simulink model "BESS_test_new"  (Simulink 8.1)
settings: Solver=ode1  StartTime=0.0  StopTime=15  FixedStep=Ts  MaxStep=1e-3  RelTol=1e-3
model workspace (MAT data in the model file):
  op_snapshot1 : opcond.OperatingPoint (value not decoded)
undefined symbols (not defined in the file or in its folder): f, H, Lgrid, Pgrid, Rgrid, RotatingMachine_lib, sampdT, sys_mech, Tc, Ts, Vgrid, VSource
libraries: powerlib x26, powerlib_meascontrol x6, transformer_lib x4, simulink x4, breaker_lib x3, Load_lib x3, cables_lib x2, BESS_lib x1, debounce_lib x1
settings Model: ARTEMISmethode_block_infos=$$__separator__$$RS/ARTEMIS Guide$$__separator__$$  Creator=RE25624  LastModifiedBy=ch24070  SimulationMode=accelerator
settings SolverCC: ZeroCrossAlgorithm=Adaptive
settings DataIOCC: ExternalInput=getinputstruct(op_snapshot1)  InitialState=getstatestruct(op_snapshot1)  LimitDataPoints=off  MaxDataPoints=90060  SignalLoggingSaveFormat=Dataset  SaveOutput=off  SignalLogging=off  DSMLogging=off  SaveTime=off  OutputSaveName=result
settings OptimizationCC: BlockReduction=off  OptimizeBlockIOStorage=off  BufferReuse=off  ExpressionFolding=off  LocalBlockOutputs=off  EfficientMapNaN2IntZero=off
settings DebuggingCC: MaxConsecutiveZCsMsg=warning  IgnoredZcDiagnostic=none  SolverPrmCheckMsg=none  MultiTaskRateTransMsg=warning  FcnCallInpInsideContextMsg=EnableAllAsWarning  UnconnectedLineMsg=none  FrameProcessingCompatibilityMsg=error  ModelReferenceExtraNoncontSigs=warning
settings HardwareCC: TargetBitPerPointer=64  TargetLongLongMode=on  TargetIntDivRoundTo=Zero  TargetEndianess=LittleEndian  TargetWordSize=64  TargetHWDeviceType=MATLAB Host  ProdEqTarget=off
settings ModelReferenceCC: UpdateModelReferenceTargets=IfOutOfDate
settings SFSimCC: SFSimEcho=off
settings CodeAppCC: MaxIdLength=128
settings GRTTargetCC: CodeReplacementLibrary=C89/C90 (ANSI)  GeneratePreprocessorConditionals=Use local settings

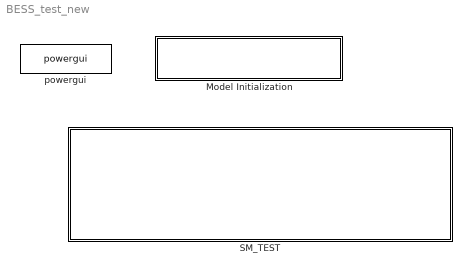
== system BESS_test_new ==
  Model Initialization : Subsystem  AncestorBlock=artemis/Tools /Misc/Model Initialization  mask(Model Functions){InitFcnX=, prel=off, posl=on, inif=on, strf=off}
      mask prompts: InitFcnX "Initialisation"; prel "Preload Function"; posl "PostLoad Function"; inif "InitFcn"; strf "StartFcn"
      mask init:
      | currentBlock = gcb;
      | root = bdroot(currentBlock);
      | 
      | if ~strcmp(get_param(root,'BlockDiagramType'),'library')
      |     if prel==1
      |         set_param(root, 'PreLoadFcn', InitFcnX);
      |     else
      |         set_param(root, 'PreLoadFcn', '');
      |     end
      |     if inif==1
      |         set_param(root, 'InitFcn', InitFcnX);
      |     else
      |         set_param(root, 'InitFcn', '');
      |     end
      |     if strf==1
      |         set_param(root, 'StartFcn', InitFcnX);
      |     else
      |         set_param(root, 'StartFcn', '');
      |     end
      |     if posl==1
      |         set_param(root, 'PostLoadFcn', InitFcnX);
      |     else
      |         set_param(root, 'PostLoadFcn', '');
      |     end
      | end
      | 
      | pos = get_param(currentBlock, 'Position');
      | width = pos(3) - pos(1); height = pos(4) - pos(2);
      | txt = [ upper(root) '\n' '- InitFcn. . . . . '  get_param(root, 'InitFcn') ];
      settings: CopyFcn=set_param(gcb,'LinkStatus','inactive')
      mask Display: text(5, height*0.5, txt, 'horizontalAlignment', 'left', 'verticalAlignment', 'middle') ;
  SM_TEST : Subsystem
  powergui : powerlib/powergui  Priority=2  SimulationMode=Discrete  SolverType=Tustin  SampleTime=Ts  frequency=60  SPID=off  DisableSnubberDevices=off  DisableRonSwitches=off  DisableVfSwitches=off  SwTol=0  DisplayEquations=off  Interpol=off  ExternalGateDelay=off  methode=off  Ts=0  FunctionMessages=off  echomessages=off  HookPort=off  EnableUseOfTLC=off  x0status=blocks  frequencyindice=0  Pbase=100e6  ErrMax=1e-4  Iterations=50  UnitsV=kV  UnitsW=MW  buscounter=0  RestoreLinks=warning  ResistiveCurrentMeasurement=off  Frange=logspace(-2,3,50)  Ylog=on  Xlog=on  ShowGrid=off  save=off  variable=ZData  structure=0  ZoomFFT=on  StartTime=0.0  cycles=2  DisplayStyle=off  fundamental=60  FreqAxis=off  MaxFrequency=1000  frequencyindicesteady=1  RmsSteady=1  display=off

== system BESS_test_new/Model Initialization ==

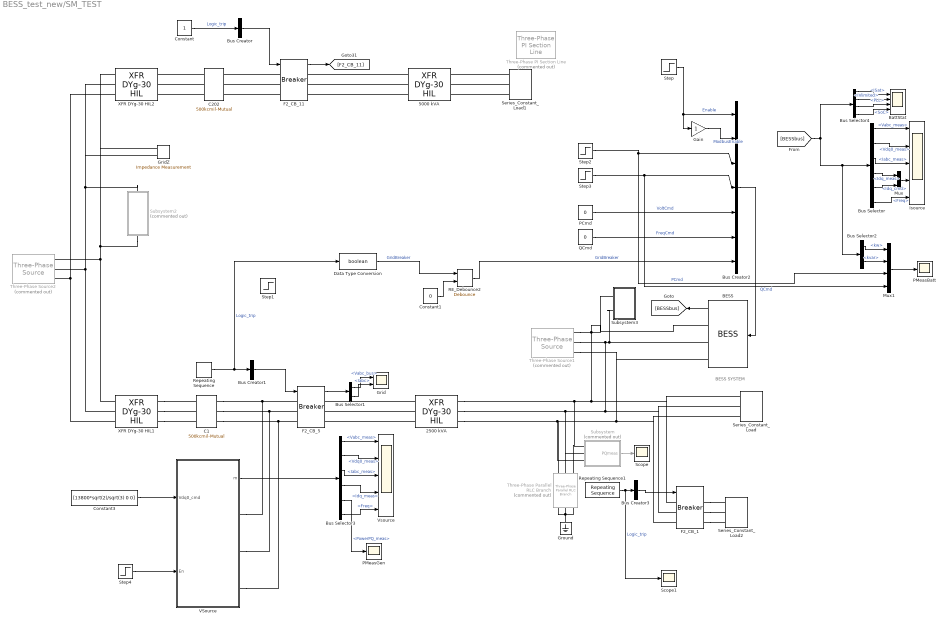
== system BESS_test_new/SM_TEST ==
  note: BESS SYSTEM
  2500 kVA : transformer_lib/XFR DYg-30 HIL  Rating=2500  Vp=13800  Vs=480  Z=5.56  XR=5.52
  5000 kVA : transformer_lib/XFR DYg-30 HIL  Rating=5000  Vp=13800  Vs=480  Z=5.50  XR=5.44
  BESS : BESS_lib/BESS
  BattStat : Scope  NumInputPorts=4
      settings: TimeRange=auto  MaxDataPoints=5000  SaveToWorkspace=off  SaveName=ScopeData2  YMin=-1.00000~-1.00000~-0.125~49.999925  YMax=1.00000~1.00000~1.125~50.000008  SampleTime=-1
  Bus Creator : BusCreator  Inputs=1
  Bus Creator1 : BusCreator  Inputs=1
  Bus Creator2 : BusCreator  Inputs=7
  Bus Creator3 : BusCreator  Inputs=1
  Bus Selector : BusSelector  OutputSignals=Inverter.Vabc_meas,Inverter.Vdq0_meas,Inverter.Iabc_meas,Inverter.Idq_meas,Inverter.Idq_cmd,Inverter.Freq
  Bus Selector1 : BusSelector  OutputSignals=Vabc_bus,Iabc
  Bus Selector2 : BusSelector  OutputSignals=Inverter.kw,Inverter.kvar
  Bus Selector3 : BusSelector  OutputSignals=Vabc_meas,Vdq0_meas,Iabc_meas,Idq_meas,PowerPQ_meas,Freq
  Bus Selector4 : BusSelector  OutputSignals=Inverter.faults.ISat,Inverter.faults.IVlimited,Inverter.faults.PLL,Battery.SoC
  C1 : cables_lib/500kcmil-Mutual  length=2000  par_sets=1  ratio=3
  C202 : cables_lib/500kcmil-Mutual  length=2000  par_sets=1  ratio=3
  Constant : Constant
  Constant1 : Constant  Value=0
  Constant3 : Constant  Value=[13800*sqrt(2)/sqrt(3) 0 0]
  Data Type Conversion : DataTypeConversion  OutDataTypeStr=boolean
  F2_CB_1 : breaker_lib/Breaker  Ts=Ts  mech_delay=3/60
  F2_CB_11 : breaker_lib/Breaker  Ts=Ts  mech_delay=3/60
  F2_CB_5 : breaker_lib/Breaker  Ts=Ts  mech_delay=3/60
  Gain : Gain
  Grid : Scope  NumInputPorts=2
      settings: TimeRange=auto  MaxDataPoints=5000  SaveToWorkspace=off  SaveName=ScopeData2  YMin=-14548.7743~-76.73519  YMax=14146.20278~74.89717  SampleTime=-1
  GridZ : powerlib/Measurements/Impedance Measurement  LConnTagsString=+|-  Factor=1
  Ground : powerlib/Elements/Ground  LConnTagsString=a
  Isource : Scope  NumInputPorts=5
      settings: TimeRange=auto  MaxDataPoints=5000  SaveName=ScopeData  YMin=-637.83955~-497.79073~-1602.05268~-1092.74993~59.90896  YMax=586.43964~568.58935~1602.13671~1545.94373~60.13357  SampleTime=-1
  Mux : Mux  Inputs=2
  Mux1 : Mux
  PCmd : Constant  Value=0
  PMeasBatt : Scope
      settings: TimeRange=auto  MaxDataPoints=5000  SaveToWorkspace=off  YMin=-1678.43829  YMax=1001.5492  SampleTime=-1
  PMeasGen : Scope
      settings: TimeRange=auto  MaxDataPoints=5000  SaveToWorkspace=off  SaveName=ScopeData2  YMin=-2639050.74714  YMax=4701504.7437  SampleTime=-1
  QCmd : Constant  Value=0
  RE_Debounce2 : debounce_lib/Debounce  Ts=sampdT  Td=0.05
  Repeating Sequence : simulink/Sources/Repeating Sequence  rep_seq_t=[0 2 2+Ts 6 6+Ts 100]  rep_seq_y=[1 1 0 0 1 1]
  Repeating Sequence1 : simulink/Sources/Repeating Sequence  rep_seq_t=[0, 4, 4+Ts, 5, 5+Ts, 8, 8+Ts 20]  rep_seq_y=[0 0 1 1 0 0 1 1]
  Scope : Scope
      settings: TimeRange=auto  MaxDataPoints=5000  SaveToWorkspace=off  YMin=-798029.94386  YMax=1422067.88409  SampleTime=-1
  Scope1 : Scope
      settings: TimeRange=auto  MaxDataPoints=5000  SaveToWorkspace=off  SaveName=ScopeData3  YMin=-0.125  YMax=1.125  SampleTime=-1
  Series_Constant_Load : Load_lib/Series_Constant_Load  v=460  kVA=400  pf=0.90
  Series_Constant_Load1 : Load_lib/Series_Constant_Load  v=460  kVA=100  pf=0.90
  Series_Constant_Load2 : Load_lib/Series_Constant_Load  v=460  kVA=300  pf=0.90
  Step : Step  Time=0.1  SampleTime=0
  Step1 : Step  Time=0.5  Before=1  After=0  SampleTime=0
  Step2 : Step  Time=13.5  After=-500  SampleTime=0
  Step3 : Step  Time=14  After=-500  SampleTime=0
  Step4 : Step  Time=0  SampleTime=0
  Subsystem : Subsystem  Commented=on  mask{V=480, P=1e3, PF=0.9}
      mask prompts: V "Nominal voltage LL"; P "P (kVA)"
      mask init:
      | Rpar = V^2/(P*1e3*PF)
      | Lpar = (V^2/((P*1e3*sqrt(1-PF^2))/3))/377
      | if Lpar == Inf
      |     Lser=0
      |     Rser=Rpar
      | else
      |     Lser = 1e-3
      |     Rser = (-Lpar^2)/(Rpar+Lpar)+Lpar-Lser
      | end
  Subsystem2 : Subsystem  Commented=on
  Subsystem3 : Subsystem
  Three-Phase PI Section Line : powerlib/Elements/Three-Phase PI Section Line  Commented=on  LConnTagsString=a|b|c  RConnTagsString=A|B|C  Frequency=60  Resistances=[ 0.01273 0.3864]  Inductances="[ 0.9337e-3  4.1264e-3]"  Capacitances=[12.74e-9 7.751e-9]  Length=100
  Three-Phase Parallel RLC Branch : powerlib/Elements/Three-Phase Parallel RLC Branch  Commented=on  LConnTagsString=A|B|C  RConnTagsString=A|B|C  BranchType=R  Resistance=Vgrid^2/(200*1e3/3);  Inductance=(Vgrid^2/((1000e3*sqrt(1-0.9^2))/3))/377  Capacitance=1e-6  Measurements=None
  Three-Phase Source1 : powerlib/Electrical Sources/Three-Phase Source  Commented=on  InternalConnection=Yg  VoltagePhases=off  Voltage=480  PhaseAngle=0  Voltage_phases=[25e3 25e3 25e3]/sqrt(3)  PhaseAngles_phases=[0 -120 +120]  Frequency=60  NonIdealSource=on  SpecifyImpedance=off  Resistance=Lgrid  Inductance=Rgrid  ShortCircuitLevel=2000e6  BaseVoltage=480  XRratio=100  BusType=swing  Pref=0  Qref=0  Prefabc=[10e3, 10e3, 10e3]  Qrefabc=[0, 0, 0]  Qmin=-inf  Qmax=inf
  Three-Phase Source2 : powerlib/Electrical Sources/Three-Phase Source  Commented=on  InternalConnection=Yg  VoltagePhases=off  Voltage=115000  PhaseAngle=0  Voltage_phases=[25e3 25e3 25e3]/sqrt(3)  PhaseAngles_phases=[0 -120 +120]  Frequency=60  NonIdealSource=on  SpecifyImpedance=on  Resistance=0.8929  Inductance=16.58e-3  ShortCircuitLevel=2000e6  BaseVoltage=115000  XRratio=100  BusType=swing  Pref=0  Qref=0  Prefabc=[10e3, 10e3, 10e3]  Qrefabc=[0, 0, 0]  Qmin=-inf  Qmax=inf
  VSource : Subsystem  AncestorBlock=RotatingMachine_lib/VSource
  Vsource : Scope  NumInputPorts=5
      settings: TimeRange=auto  MaxDataPoints=5000  YMin=-14095.34302~-1426.98059~-258.17624~-157.47216~59.97105  YMax=14085.47927~12733.83164~249.33503~278.13701~60.01653  SampleTime=-1
  XFR DYg-30 HIL1 : transformer_lib/XFR DYg-30 HIL  Rating=50000  Vp=115000  Vs=13800  Z=6  XR=30
  XFR DYg-30 HIL2 : transformer_lib/XFR DYg-30 HIL  Rating=50000  Vp=115000  Vs=13800  Z=6  XR=30
  wires:
  F2_CB_5/1 -> Bus Selector1/1
  F2_CB_11/1 -> [F2_CB_11]
  Constant/1 -> Bus Creator/1  "Logic_trip"
  Repeating Sequence/1 -> Data Type Conversion/1, Bus Creator1/1  "Logic_trip"
  Bus Creator1/1 -> F2_CB_5/1
  Bus Creator/1 -> F2_CB_11/1
  Step/1 -> Gain/1, Bus Creator2/1  "Enable"
  Step2/1 -> Mux1/3, Bus Creator2/3  "PCmd"
  Step3/1 -> Mux1/4, Bus Creator2/4  "QCmd"
  Bus Creator2/1 -> BESS/1
  Bus Selector/6 -> Isource/5  "<Freq>"
  Bus Selector/3 -> Isource/3  "<Iabc_meas>"
  Bus Selector/1 -> Isource/1  "<Vabc_meas>"
  Bus Selector/2 -> Isource/2  "<Vdq0_meas>"
  Subsystem/1(PQmeas) -> Scope/1
  Bus Selector1/1 -> Grid/1  "<Vabc_bus>"
  Bus Selector1/2 -> Grid/2  "<Iabc>"
  Mux/1 -> Isource/4
  Bus Selector/4 -> Mux/1  "<Idq_meas>"
  Bus Selector/5 -> Mux/2  "<Idq_cmd>"
  BESS/1 -> [BESSbus]
  [BESSbus] -> Bus Selector/1, Bus Selector2/1, Bus Selector4/1
  Bus Selector2/1 -> Mux1/1  "<kw>"
  Mux1/1 -> PMeasBatt/1
  Repeating Sequence1/1 -> Scope1/1, Bus Creator3/1  "Logic_trip"
  Bus Creator3/1 -> F2_CB_1/1
  Constant3/1 -> VSource/1(Vdq0_cmd)
  Step4/1 -> VSource/2(En)
  Bus Selector3/3 -> Vsource/3  "<Iabc_meas>"
  Bus Selector3/1 -> Vsource/1  "<Vabc_meas>"
  Bus Selector3/2 -> Vsource/2  "<Vdq0_meas>"
  Bus Selector3/4 -> Vsource/4  "<Idq_meas>"
  VSource/1(m) -> Bus Selector3/1
  Bus Selector3/6 -> Vsource/5  "<Freq>"
  Bus Selector3/5 -> PMeasGen/1  "<PowerPQ_meas>"
  Gain/1 -> Bus Creator2/2  "ModbusEnable"
  Bus Selector2/2 -> Mux1/2  "<kvar>"
  Bus Selector4/2 -> BattStat/2  "<IVlimited>"
  Bus Selector4/1 -> BattStat/1  "<ISat>"
  Bus Selector4/3 -> BattStat/3  "<PLL>"
  PCmd/1 -> Bus Creator2/5  "VoltCmd"
  QCmd/1 -> Bus Creator2/6  "FreqCmd"
  RE_Debounce2/1 -> Bus Creator2/7  "GridBreaker"
  Bus Selector4/4 -> BattStat/4  "<SoC>"
  Constant1/1 -> RE_Debounce2/2
  Data Type Conversion/1 -> RE_Debounce2/1  "GridBreaker"
  connections:
  5000 kVA/LConn2 -- F2_CB_11/RConn2
  2500 kVA/LConn1 -- F2_CB_5/RConn1
  2500 kVA/LConn3 -- F2_CB_5/RConn3
  2500 kVA/LConn2 -- F2_CB_5/RConn2
  5000 kVA/LConn1 -- F2_CB_11/RConn1
  5000 kVA/LConn3 -- F2_CB_11/RConn3
  2500 kVA/RConn1 -- BESS/RConn1 -- Subsystem3/LConn1 -- Three-Phase Source1/RConn1 -- F2_CB_1/LConn1 -- Series_Constant_Load/LConn1 -- Three-Phase Parallel RLC Branch/LConn3 -- Subsystem/LConn1
  2500 kVA/RConn3 -- BESS/RConn3 -- Three-Phase Source1/RConn3 -- F2_CB_1/LConn3 -- Series_Constant_Load/LConn3 -- Three-Phase Parallel RLC Branch/LConn1 -- Subsystem/LConn3
  XFR DYg-30 HIL1/LConn1 -- GridZ/LConn1 -- XFR DYg-30 HIL2/LConn1 -- Subsystem2/LConn1 -- Three-Phase Source2/RConn1
  XFR DYg-30 HIL1/LConn2 -- GridZ/LConn2 -- XFR DYg-30 HIL2/LConn2 -- Subsystem2/RConn1 -- Three-Phase Source2/RConn2
  XFR DYg-30 HIL1/LConn3 -- XFR DYg-30 HIL2/LConn3 -- Three-Phase Source2/RConn3
  Series_Constant_Load1/LConn3 -- 5000 kVA/RConn3
  Series_Constant_Load1/LConn2 -- 5000 kVA/RConn2
  Series_Constant_Load1/LConn1 -- 5000 kVA/RConn1
  C202/LConn1 -- XFR DYg-30 HIL2/RConn1
  C202/LConn2 -- XFR DYg-30 HIL2/RConn2
  C202/LConn3 -- XFR DYg-30 HIL2/RConn3
  XFR DYg-30 HIL1/RConn1 -- C1/LConn1
  XFR DYg-30 HIL1/RConn2 -- C1/LConn2
  XFR DYg-30 HIL1/RConn3 -- C1/LConn3
  C1/RConn2 -- VSource/RConn2 -- F2_CB_5/LConn2
  C1/RConn1 -- VSource/RConn1 -- F2_CB_5/LConn1
  C1/RConn3 -- VSource/RConn3 -- F2_CB_5/LConn3
  F2_CB_11/LConn1 -- C202/RConn1
  F2_CB_11/LConn2 -- C202/RConn2
  F2_CB_11/LConn3 -- C202/RConn3
  Ground/LConn1 -- Three-Phase Parallel RLC Branch/RConn3 -- Three-Phase Parallel RLC Branch/RConn1 -- Three-Phase Parallel RLC Branch/RConn2
  F2_CB_1/RConn1 -- Series_Constant_Load2/LConn1
  F2_CB_1/RConn2 -- Series_Constant_Load2/LConn2
  F2_CB_1/RConn3 -- Series_Constant_Load2/LConn3
  Subsystem3/LConn2 -- BESS/RConn2 -- 2500 kVA/RConn2 -- Three-Phase Parallel RLC Branch/LConn2 -- Subsystem/LConn2 -- F2_CB_1/LConn2 -- Series_Constant_Load/LConn2 -- Three-Phase Source1/RConn2

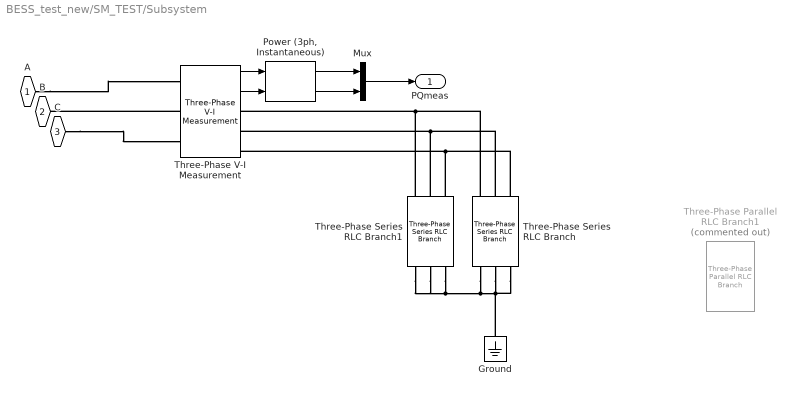
== system BESS_test_new/SM_TEST/Subsystem ==
  Ground : powerlib/Elements/Ground  LConnTagsString=a
  Mux : Mux  Inputs=2
  "Power (3ph, Instantaneous)" : powerlib_meascontrol/Measurements/Power (3ph, Instantaneous)
  Three-Phase Parallel RLC Branch1 : powerlib/Elements/Three-Phase Parallel RLC Branch  Commented=on  LConnTagsString=A|B|C  RConnTagsString=A|B|C  BranchType=RL  Resistance=Vgrid^2/(1000e3*0.9/3)  Inductance=(Vgrid^2/((1000e3*sqrt(1-0.9^2))/3))/377  Capacitance=1e-6  Measurements=None
  Three-Phase Series RLC Branch : powerlib/Elements/Three-Phase Series RLC Branch  LConnTagsString=A|B|C  RConnTagsString=A|B|C  BranchType=L  Resistance=Rser  Inductance=Lpar  Capacitance=1e-6  Measurements=None
  Three-Phase Series RLC Branch1 : powerlib/Elements/Three-Phase Series RLC Branch  LConnTagsString=A|B|C  RConnTagsString=A|B|C  BranchType=R  Resistance=Rpar  Inductance=Lser  Capacitance=1e-6  Measurements=None
  Three-Phase V-I Measurement : powerlib/Measurements/Three-Phase V-I Measurement  VoltageMeasurement=phase-to-ground  SetLabelV=off  LabelV=Vabc  Vpu=off  VpuLL=off  CurrentMeasurement=yes  SetLabelI=off  LabelI=Iabc  Ipu=off  Pbase=100e6  Vbase=500e3  OutputType=Complex  PhasorSimulation=off  PSBequivalent=0
  A : PMIOPort  Port=1  Side=Left
  B : PMIOPort  Port=2  Side=Left
  C : PMIOPort  Port=3  Side=Left
  PQmeas : Outport
  wires:
  Three-Phase V-I Measurement/1 -> "Power (3ph, Instantaneous)"/1
  Three-Phase V-I Measurement/2 -> "Power (3ph, Instantaneous)"/2
  "Power (3ph, Instantaneous)"/1 -> Mux/1
  "Power (3ph, Instantaneous)"/2 -> Mux/2
  Mux/1 -> PQmeas/1
  connections:
  Three-Phase V-I Measurement/LConn2 -- B/RConn1
  C/RConn1 -- Three-Phase V-I Measurement/LConn3
  A/RConn1 -- Three-Phase V-I Measurement/LConn1
  Three-Phase Series RLC Branch/LConn1 -- Three-Phase Series RLC Branch1/LConn1 -- Three-Phase V-I Measurement/RConn1
  Three-Phase Series RLC Branch/LConn2 -- Three-Phase Series RLC Branch1/LConn2 -- Three-Phase V-I Measurement/RConn2
  Three-Phase Series RLC Branch/LConn3 -- Three-Phase Series RLC Branch1/LConn3 -- Three-Phase V-I Measurement/RConn3
  Ground/LConn1 -- Three-Phase Series RLC Branch1/RConn3 -- Three-Phase Series RLC Branch1/RConn2 -- Three-Phase Series RLC Branch1/RConn1 -- Three-Phase Series RLC Branch/RConn1 -- Three-Phase Series RLC Branch/RConn2 -- Three-Phase Series RLC Branch/RConn3

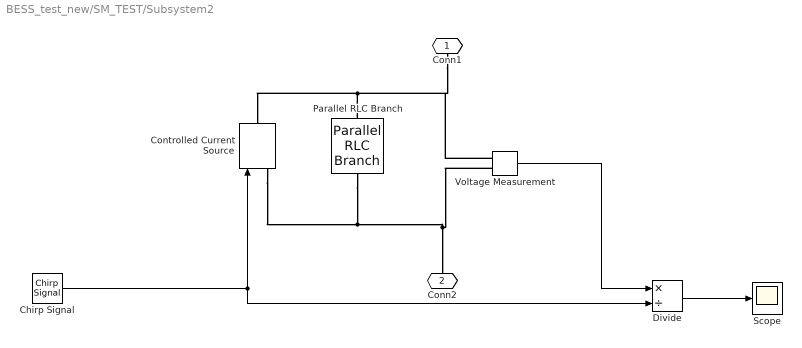
== system BESS_test_new/SM_TEST/Subsystem2 ==
  Chirp Signal : simulink/Sources/Chirp Signal  f1=0.1  T=1  f2=1000
  Controlled Current Source : powerlib/Electrical Sources/Controlled Current Source  Initialize=on  Source_Type=AC  Amplitude=0  Phase=0  Frequency=0  Measurements=None
  Divide : Product  Inputs=*/
  Parallel RLC Branch : powerlib/Elements/Parallel RLC Branch  LConnTagsString=a  RConnTagsString=__new0  BranchType=R  Resistance=1e6  Inductance=1e-3  SetiL0=off  InitialCurrent=0  Capacitance=1e-6  Setx0=off  InitialVoltage=0  Measurements=None
  Scope : Scope
      settings: TimeRange=auto  MaxDataPoints=5000  SaveToWorkspace=off  YMin=-88482354.99366  YMax=99069686.1974  SampleTime=-1
  Voltage Measurement : powerlib/Measurements/Voltage Measurement  PhasorSimulation=off  OutputType=Complex  PSBequivalent=0
  Conn1 : PMIOPort  Port=1  Side=Right
  Conn2 : PMIOPort  Port=2  Side=Left
  wires:
  Chirp Signal/1 -> Divide/2, Controlled Current Source/1
  Voltage Measurement/1 -> Divide/1
  Divide/1 -> Scope/1
  connections:
  Controlled Current Source/LConn1 -- Parallel RLC Branch/RConn1 -- Voltage Measurement/LConn2 -- Conn2/RConn1
  Parallel RLC Branch/LConn1 -- Conn1/RConn1 -- Voltage Measurement/LConn1 -- Controlled Current Source/RConn1

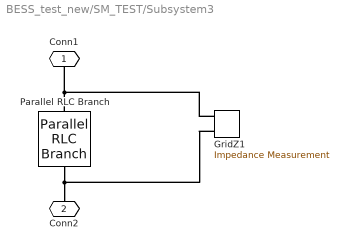
== system BESS_test_new/SM_TEST/Subsystem3 ==
  GridZ1 : powerlib/Measurements/Impedance Measurement  LConnTagsString=+|-  Factor=1
  Parallel RLC Branch : powerlib/Elements/Parallel RLC Branch  LConnTagsString=a  RConnTagsString=__new0  BranchType=R  Resistance=1e6  Inductance=1e-3  SetiL0=off  InitialCurrent=0  Capacitance=1e-6  Setx0=off  InitialVoltage=0  Measurements=None
  Conn1 : PMIOPort  Port=1  Side=Left
  Conn2 : PMIOPort  Port=2  Side=Left
  connections:
  GridZ1/LConn1 -- Parallel RLC Branch/LConn1 -- Conn1/RConn1
  GridZ1/LConn2 -- Parallel RLC Branch/RConn1 -- Conn2/RConn1

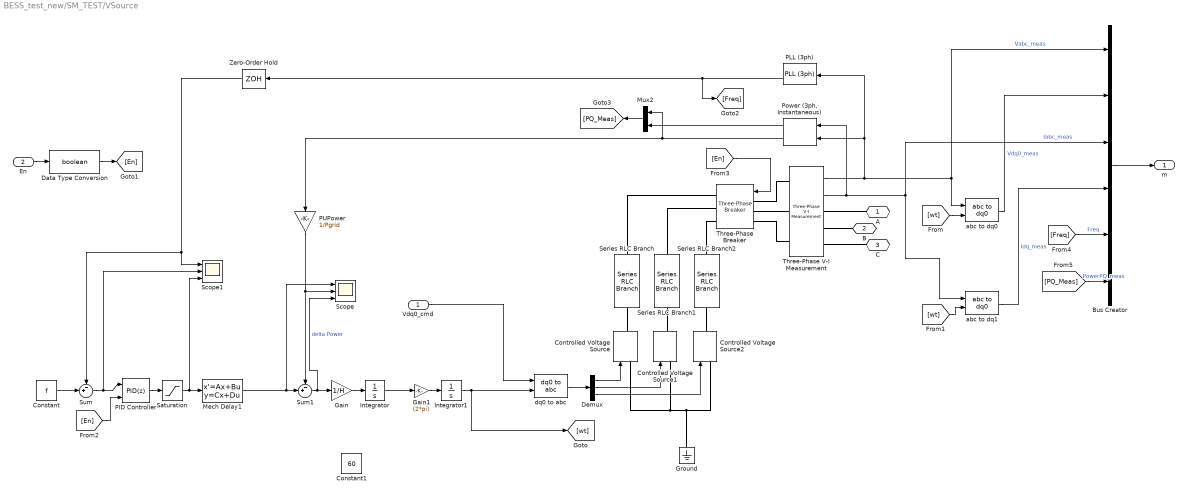
== system BESS_test_new/SM_TEST/VSource ==
  Vdq0_cmd : Inport
  En : Inport  Port=2
  Bus Creator : BusCreator  Inputs=6
  Constant : Constant  Value=f
  Constant1 : Constant  Value=60
  Controlled Voltage Source : powerlib/Electrical Sources/Controlled Voltage Source  Initialize=on  Source_Type=AC  Amplitude=0  Phase=0  Frequency=0  Measurements=None
  Controlled Voltage Source1 : powerlib/Electrical Sources/Controlled Voltage Source  Initialize=on  Source_Type=AC  Amplitude=0  Phase=0  Frequency=0  Measurements=None
  Controlled Voltage Source2 : powerlib/Electrical Sources/Controlled Voltage Source  Initialize=on  Source_Type=AC  Amplitude=0  Phase=0  Frequency=0  Measurements=None
  Data Type Conversion : DataTypeConversion  OutDataTypeStr=boolean
  Demux : Demux  Outputs=3
  Gain : Gain  Gain=1/H
  Gain1 : Gain  Gain=(2*pi)
  Ground : powerlib/Elements/Ground  LConnTagsString=a
  Integrator : Integrator  InitialCondition=f
  Integrator1 : Integrator
  Mech Delay1 : StateSpace  A=sys_mech.A  B=sys_mech.B  C=sys_mech.C  D=sys_mech.D  X0=0.3/sys_mech.C
  Mux2 : Mux  Inputs=2
  PID Controller : simulink/Continuous/PID Controller  Controller=PID  TimeDomain=Discrete-time  SampleTime=Tc  IntegratorMethod=Forward Euler  FilterMethod=Forward Euler  Form=Parallel  UseFilter=on  ControllerParametersSource=internal  P=10.7070638462033  I=6.52954426447568  D=2.34676955636377  N=24.9126202349528  InitialConditionSource=internal  InitialConditionForIntegrator=0.1  InitialConditionForFilter=0  ExternalReset=level  LimitOutput=off  UpperSaturationLimit=inf  LowerSaturationLimit=-inf  LinearizeAsGain=on  AntiWindupMode=none  Kb=1  TrackingMode=off  Kt=1  PParamMin=[]  PParamMax=[]  IParamMin=[]  IParamMax=[]  DParamMin=[]  DParamMax=[]  NParamMin=[]  NParamMax=[]  KbParamMin=[]  KbParamMax=[]  KtParamMin=[]  KtParamMax=[]  POutMin=[]  POutMax=[]  IOutMin=[]  IOutMax=[]  DOutMin=[]  DOutMax=[]  NOutMin=[]  NOutMax=[]  KbOutMin=[]  KbOutMax=[]  KtOutMin=[]  KtOutMax=[]  IntegratorOutMin=[]  IntegratorOutMax=[]  FilterOutMin=[]  FilterOutMax=[]  SumOutMin=[]  SumOutMax=[]  SumI1OutMin=[]  SumI1OutMax=[]  SumI2OutMin=[]  SumI2OutMax=[]  SumI3OutMin=[]  SumI3OutMax=[]  SumDOutMin=[]  SumDOutMax=[]  SaturationOutMin=[]  SaturationOutMax=[]  IntegratorContinuousStateAttributes=''  IntegratorStateMustResolveToSignalObject=off  IntegratorRTWStateStorageClass=Auto  FilterContinuousStateAttributes=''  FilterStateMustResolveToSignalObject=off  FilterRTWStateStorageClass=Auto  DifferentiatorICPrevScaledInput=0  DifferentiatorOutMin=[]  DifferentiatorOutMax=[]
  PLL (3ph) : powerlib_meascontrol/PLL/PLL (3ph)  Fmin=45  Par_Init=[0, 60]  ParK=[180, 3200, 1]  TcD=1e-4  MaxRateChangeFreq=1200  FilterCutOffFreq=25  Ts=0  AGC=on
  PUPower : Gain  Gain=1/Pgrid
  "Power (3ph, Instantaneous)" : powerlib_meascontrol/Measurements/Power (3ph, Instantaneous)
  Saturation : Saturate  UpperLimit=1.2  LowerLimit=0
  Scope : Scope  NumInputPorts=3
      settings: TimeRange=auto  MaxDataPoints=5000  SaveToWorkspace=off  SaveName=ScopeData3  YMin=0.0899~-0.60777~-5.51951  YMax=0.32334~5.65357~0.78328  SampleTime=-1
  Scope1 : Scope  NumInputPorts=3
      settings: TimeRange=auto  MaxDataPoints=5000  SaveToWorkspace=off  SaveName=ScopeData4  YMin=59.89374~-0.07085~-0.15  YMax=60.07033~0.18183~1.35  SampleTime=-1
  Series RLC Branch : powerlib/Elements/Series RLC Branch  LConnTagsString=__new0  RConnTagsString=__new0  BranchType=RL  Resistance=Rgrid  Inductance=Lgrid  SetiL0=off  InitialCurrent=0  Capacitance=0  Setx0=off  InitialVoltage=0  Measurements=None
  Series RLC Branch1 : powerlib/Elements/Series RLC Branch  LConnTagsString=__new0  RConnTagsString=__new0  BranchType=RL  Resistance=Rgrid  Inductance=Lgrid  SetiL0=off  InitialCurrent=0  Capacitance=0  Setx0=off  InitialVoltage=0  Measurements=None
  Series RLC Branch2 : powerlib/Elements/Series RLC Branch  LConnTagsString=__new0  RConnTagsString=__new0  BranchType=RL  Resistance=Rgrid  Inductance=Lgrid  SetiL0=off  InitialCurrent=0  Capacitance=0  Setx0=off  InitialVoltage=0  Measurements=None
  Sum : Sum  Inputs=-+|
  Sum1 : Sum  Inputs=-+|
  Three-Phase V-I Measurement : powerlib/Measurements/Three-Phase V-I Measurement  VoltageMeasurement=phase-to-ground  SetLabelV=off  LabelV=Vabc  Vpu=off  VpuLL=off  CurrentMeasurement=yes  SetLabelI=off  LabelI=Iabc  Ipu=off  Pbase=100e6  Vbase=500e3  OutputType=Complex  PhasorSimulation=off  PSBequivalent=0
  Three-Phase Breaker : powerlib/Elements/Three-Phase Breaker  InitialState=open  SwitchA=on  SwitchB=on  SwitchC=on  SwitchTimes="[1/60  5/60]"  External=on  BreakerResistance=0.01  SnubberResistance=1e6  SnubberCapacitance=inf  Measurements=None
  Zero-Order Hold : ZeroOrderHold  SampleTime=Tc
  abc to dq0 : powerlib_meascontrol/Transformations/abc to dq0  Alignment=90 degrees behind phase A axis
  abc to dq1 : powerlib_meascontrol/Transformations/abc to dq0  Alignment=90 degrees behind phase A axis
  dq0 to abc : powerlib_meascontrol/Transformations/dq0 to abc  Alignment=90 degrees behind phase A axis
  A : PMIOPort  Port=1  Side=Right
  B : PMIOPort  Port=2  Side=Right
  C : PMIOPort  Port=3  Side=Right
  m : Outport
  wires:
  Mux2/1 -> [PQ_Meas]
  "Power (3ph, Instantaneous)"/2 -> Mux2/2
  Bus Creator/1 -> m/1
  [Freq] -> Bus Creator/5  "Freq"
  abc to dq0/1 -> Bus Creator/2  "Vdq0_meas"
  Three-Phase V-I Measurement/2 -> abc to dq1/1, Bus Creator/3, "Power (3ph, Instantaneous)"/2  "Iabc_meas"
  Three-Phase V-I Measurement/1 -> abc to dq0/1, Bus Creator/1, "Power (3ph, Instantaneous)"/1, PLL (3ph)/1  "Vabc_meas"
  abc to dq1/1 -> Bus Creator/4  "Idq_meas"
  [PQ_Meas] -> Bus Creator/6  "PowerPQ_meas"
  [En] -> Three-Phase Breaker/1
  [En] -> PID Controller/2
  Data Type Conversion/1 -> [En]
  En/1 -> Data Type Conversion/1
  Constant/1 -> Sum/2
  PUPower/1 -> Sum1/1, Scope/2
  Mech Delay1/1 -> Sum1/2, Scope/1
  PID Controller/1 -> Saturation/1
  Saturation/1 -> Mech Delay1/1, Scope1/3
  Zero-Order Hold/1 -> Scope1/1, Sum/1
  PLL (3ph)/1 -> Zero-Order Hold/1, [Freq]
  Gain1/1 -> Integrator1/1
  "Power (3ph, Instantaneous)"/1 -> PUPower/1, Mux2/1
  Gain/1 -> Integrator/1
  Sum1/1 -> Gain/1, Scope/3  "delta Power"
  Sum/1 -> Scope1/2, PID Controller/1
  Demux/3 -> Controlled Voltage Source2/1
  Demux/2 -> Controlled Voltage Source1/1
  dq0 to abc/1 -> Demux/1
  Demux/1 -> Controlled Voltage Source/1
  Vdq0_cmd/1 -> dq0 to abc/1
  Integrator1/1 -> [wt], dq0 to abc/2
  Integrator/1 -> Gain1/1
  [wt] -> abc to dq0/2
  [wt] -> abc to dq1/2
  connections:
  Three-Phase Breaker/RConn3 -- Series RLC Branch2/LConn1
  Three-Phase Breaker/RConn2 -- Series RLC Branch1/LConn1
  Three-Phase Breaker/RConn1 -- Series RLC Branch/LConn1
  Three-Phase Breaker/LConn3 -- Three-Phase V-I Measurement/LConn3
  Three-Phase Breaker/LConn1 -- Three-Phase V-I Measurement/LConn1
  Three-Phase Breaker/LConn2 -- Three-Phase V-I Measurement/LConn2
  Controlled Voltage Source/LConn1 -- Controlled Voltage Source1/LConn1 -- Controlled Voltage Source2/LConn1 -- Ground/LConn1
  Controlled Voltage Source2/RConn1 -- Series RLC Branch2/RConn1
  Controlled Voltage Source1/RConn1 -- Series RLC Branch1/RConn1
  Controlled Voltage Source/RConn1 -- Series RLC Branch/RConn1
  Three-Phase V-I Measurement/RConn2 -- B/RConn1
  Three-Phase V-I Measurement/RConn1 -- A/RConn1
  Three-Phase V-I Measurement/RConn3 -- C/RConn1
